simulink model "PMDC_OPEN_LOOP_1"  (R2022a)
settings: Solver=VariableStepAuto  StartTime=0.0  StopTime=10.0  RelTol=1e-3
model workspace (MAT data in the model file):
  B = 0.01
  R = 0.5
  Tb = 20
  V = 160
  kb = 1.6
  kt = 1.6
  tau_a = 0.2
  tau_m = 500
settings Model: Creator=venka  LastModifiedBy=venka
settings DebuggingCC: UnconnectedInputMsg=warning  UnconnectedOutputMsg=warning  UnconnectedLineMsg=warning
settings RTWCC: DLArmComputeVersion=19.05

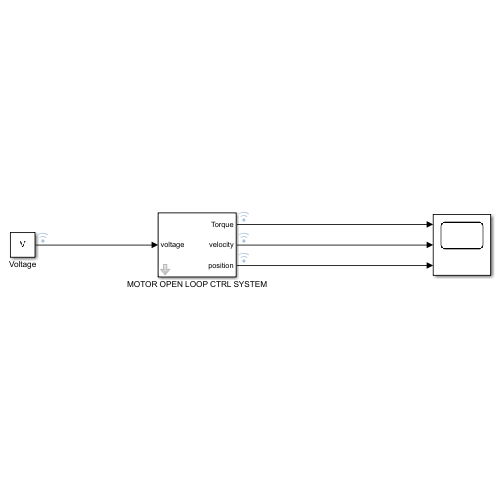
[thumbnail: Simulink's stored preview of the top-level diagram]
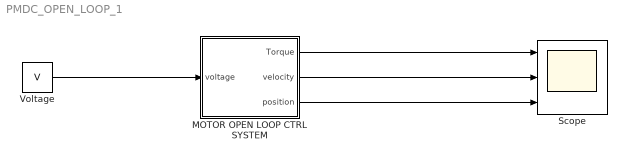
== system PMDC_OPEN_LOOP_1 ==
  MOTOR OPEN LOOP CTRL SYSTEM : Subsystem  mask{B=0.01, J=5, kb=1.6, kt=1.6, R=0.5, tau_a=0.2, tau_m=500, Tb=20, L=0.1, Parameter10=0}
      mask prompts: B "damping const"; J "inertia"; kb "back emf const"; kt "torque const"; R "Resistance"; tau_a "Electrical time const"; tau_m "Mechanical time const"; Tb "load torque"; L "Inductance"
  Scope : Scope  NumInputPorts=3
  Voltage : Constant  Value=V  mask{V=100}
      mask prompts: V "voltage"
  wires:
  Voltage/1 -> MOTOR OPEN LOOP CTRL SYSTEM/1(voltage)
  MOTOR OPEN LOOP CTRL SYSTEM/2(velocity) -> Scope/2
  MOTOR OPEN LOOP CTRL SYSTEM/3(position) -> Scope/3
  MOTOR OPEN LOOP CTRL SYSTEM/1(Torque) -> Scope/1

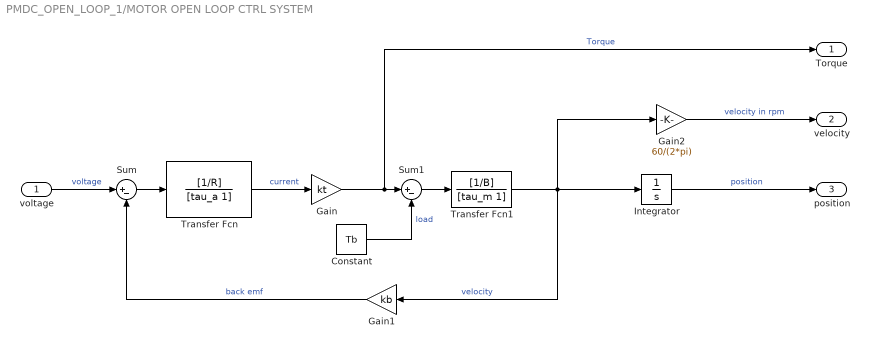
== system PMDC_OPEN_LOOP_1/MOTOR OPEN LOOP CTRL SYSTEM ==
  voltage : Inport
  Constant : Constant  Value=Tb
  Gain : Gain  Gain=kt
  Gain1 : Gain  Gain=kb
  Gain2 : Gain  Gain=60/(2*pi)
  Integrator : Integrator
  Sum : Sum  Inputs=|+-
  Sum1 : Sum  Inputs=|+-
  Transfer Fcn : TransferFcn  Numerator=[1/R]  Denominator=[tau_a 1]
  Transfer Fcn1 : TransferFcn  Numerator=[1/B]  Denominator=[tau_m 1]
  Torque : Outport
  velocity : Outport  Port=2
  position : Outport  Port=3
  wires:
  Transfer Fcn1/1 -> Integrator/1, Gain2/1, Gain1/1  "velocity"
  Gain/1 -> Torque/1, Sum1/1  "Torque"
  Gain1/1 -> Sum/2  "back emf"
  Sum/1 -> Transfer Fcn/1
  Transfer Fcn/1 -> Gain/1  "current"
  Constant/1 -> Sum1/2  "load"
  Sum1/1 -> Transfer Fcn1/1
  Integrator/1 -> position/1  "position"
  voltage/1 -> Sum/1  "voltage"
  Gain2/1 -> velocity/1  "velocity in rpm"
